simulink model "LPCtest"  (R2025a)
settings: Solver=VariableStepAuto  StartTime=0.0  StopTime=10.0  RelTol=1e-3
undefined symbols (not defined in the file): effMod_LPC, eta_lpc_map, PR_lpc_map, speed_vec_lpc, Wc_core, Wc_lpc_bp
settings Model: Creator=ramch  LastModifiedBy=ramch

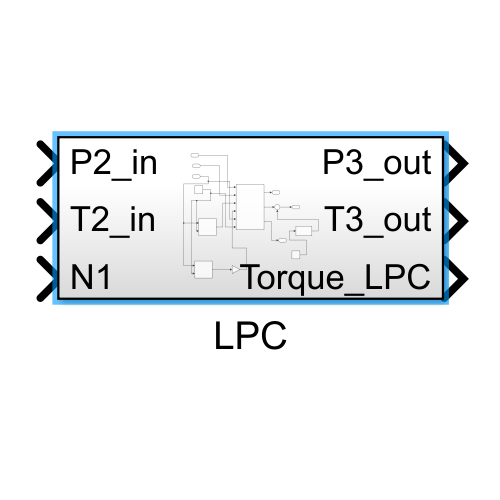
[thumbnail: Simulink's stored preview of the top-level diagram]
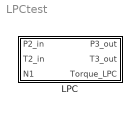
== system LPCtest ==
  LPC : Subsystem

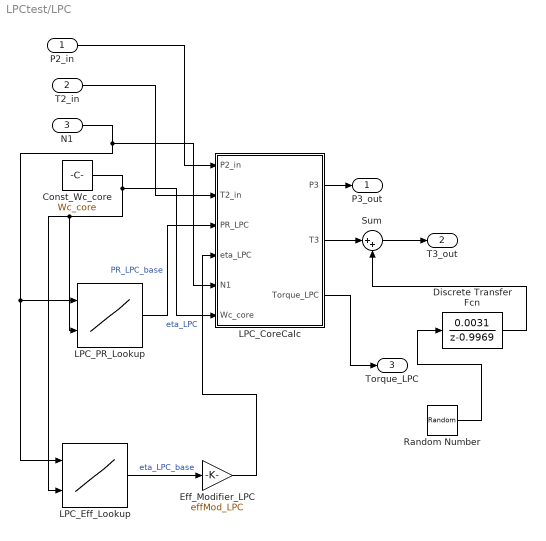
== system LPCtest/LPC ==
  P2_in : Inport
  T2_in : Inport  Port=2
  N1 : Inport  Port=3
  Const_Wc_core : Constant  Value=Wc_core
  Discrete Transfer Fcn : DiscreteTransferFcn  Numerator=0.0031  Denominator=1 -0.9969  InitialStates=0.001
  Eff_Modifier_LPC : Gain  Gain=effMod_LPC
  LPC_CoreCalc : MATLAB Function  TreatAsAtomicUnit=on
  LPC_Eff_Lookup : Lookup_n-D  BreakpointsForDimension1=speed_vec_lpc  BreakpointsForDimension2=Wc_lpc_bp  Table=eta_lpc_map  InternalRulePriority=Speed  RndMeth=Simplest
      settings: InputPortMap=u0,u1
  LPC_PR_Lookup : Lookup_n-D  BreakpointsForDimension1=speed_vec_lpc  BreakpointsForDimension2=Wc_lpc_bp  Table=PR_lpc_map  InternalRulePriority=Speed  RndMeth=Simplest
      settings: InputPortMap=u0,u1
  Random Number : RandomNumber  Variance=(0.5)  SampleTime=0.001
  Sum : Sum  Inputs=|++
  P3_out : Outport
  T3_out : Outport  Port=2
  Torque_LPC : Outport  Port=3
  wires:
  N1/1 -> LPC_CoreCalc/5(N1), LPC_Eff_Lookup/1, LPC_PR_Lookup/1
  Const_Wc_core/1 -> LPC_CoreCalc/6(Wc_core), LPC_Eff_Lookup/2, LPC_PR_Lookup/2
  LPC_Eff_Lookup/1 -> Eff_Modifier_LPC/1  "eta_LPC_base"
  P2_in/1 -> LPC_CoreCalc/1(P2_in)
  T2_in/1 -> LPC_CoreCalc/2(T2_in)
  LPC_PR_Lookup/1 -> LPC_CoreCalc/3(PR_LPC)  "PR_LPC_base"
  Eff_Modifier_LPC/1 -> LPC_CoreCalc/4(eta_LPC)  "eta_LPC"
  LPC_CoreCalc/1(P3) -> P3_out/1
  LPC_CoreCalc/3(Torque_LPC) -> Torque_LPC/1
  LPC_CoreCalc/2(T3) -> Sum/1
  Sum/1 -> T3_out/1
  Random Number/1 -> Discrete Transfer Fcn/1
  Discrete Transfer Fcn/1 -> Sum/2

== matlab function LPCtest/LPC/LPC_CoreCalc ==
  data: P2_in input; P3 output; T2_in input; PR_LPC input; eta_LPC input; N1 input; Wc_core input; T3 output; Torque_LPC output
function [P3, T3, Torque_LPC] = LPC_CoreCalc(P2_in, T2_in, PR_LPC, eta_LPC, N1, Wc_core)
% Computes LPC outlet total pressure/temperature and torque on N1

    % Constants
    gamma = 1.4;    % for air
    cp = 1004;      % J/(kg·K)

    % 1) Outlet pressure
    P3 = P2_in * PR_LPC;

    % 2) Outlet temperature (isentropic with efficiency)
    T3 = T2_in * (1 + (1/eta_LPC) * (PR_LPC^((gamma-1)/gamma) - 1));

    % 3) Convert N1 [RPM] to rad/s
    omega1 = N1 * 2 * pi / 60;

    % 4) Recover actual core mass flow from corrected Wc_core:
    Tref = 288.15;
    Pref = 101325;
    m_dot_core = Wc_core * sqrt(T2_in/Tref) * (P2_in/Pref);  % [kg/s]

    % 5) Enthalpy rise (cp * ΔT)
    delta_h_core = cp * (T3 - T2_in);

    % 6) Torque on N1 shaft due to LPC (core only)
    Torque_LPC = (m_dot_core * delta_h_core) / omega1;
end
